simulink model "TareaIntegradora"  (R2023b)
settings: Solver=VariableStepAuto  StartTime=0.0  StopTime=9  FixedStep=0.001  RelTol=1e-3  EnableMultiTasking=on
InitFcn:
  | L= 0.000938
  | J=0.0072
  | B=0.000389
  | b=B
  | R=5.2
  | km=0.5931
  | K=km
  | Radio=0.05
settings Model: ExtModeTrigDuration=2  Creator=jaime  LastModifiedBy=jaime
settings OptimizationCC: EnhancedBackFolding=on  PassReuseOutputArgsAs=Individual arguments  ZeroExternalMemoryAtStartup=off  ZeroInternalMemoryAtStartup=off  MaxStackSize=64  OptimizeBlockOrder=speed  DifferentSizesBufferReuse=on  OptimizationCustomize=off  EfficientTunableParamExpr=on
settings DebuggingCC: ParameterTunabilityLossMsg=error
settings HardwareCC: ProdBitPerInt=16  ProdBitPerPointer=16  ProdBitPerSizeT=16  ProdBitPerPtrDiffT=16  ProdLargestAtomicFloat=None  ProdWordSize=8  ProdHWDeviceType=Atmel->AVR  UseEmbeddedCoderFeatures=off
settings SFSimCC: MATLABDynamicMemAlloc=off
settings RTWCC: Description=Embedded Coder  SystemTargetFile=ert.tlc  HardwareBoard=Arduino Mega 2560  TemplateMakefile=ert_default_tmf  Toolchain=Arduino AVR  BuildConfiguration=Faster Runs
settings CodeAppCC: ForceParamTrailComments=on  IgnoreCustomStorageClasses=off  OperatorAnnotations=on  SimulinkDataObjDesc=on  SFDataObjDesc=on  InsertBlockDesc=on
settings ERTTargetCC: SupportContinuousTime=on  SupportNonInlinedSFcns=on  SupportVariableSizeSignals=on  ExtModeTransport=3  ExtModeStaticAlloc=on  ExtModeAutomaticAllocSize=off  ExtModeStaticAllocSize=2048  ExtModeMexFile=ext_xcp  ExtModeIntrfLevel=Level2 - Open

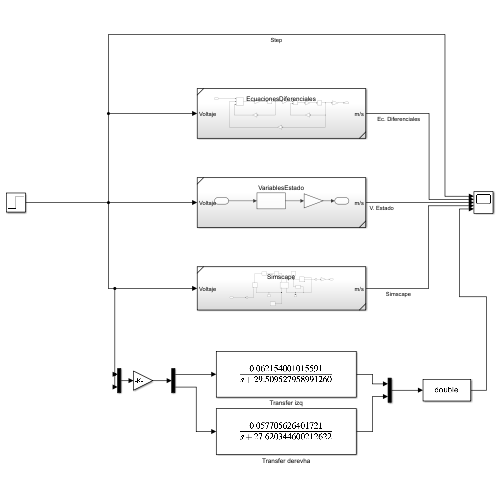
[thumbnail: Simulink's stored preview of the top-level diagram]
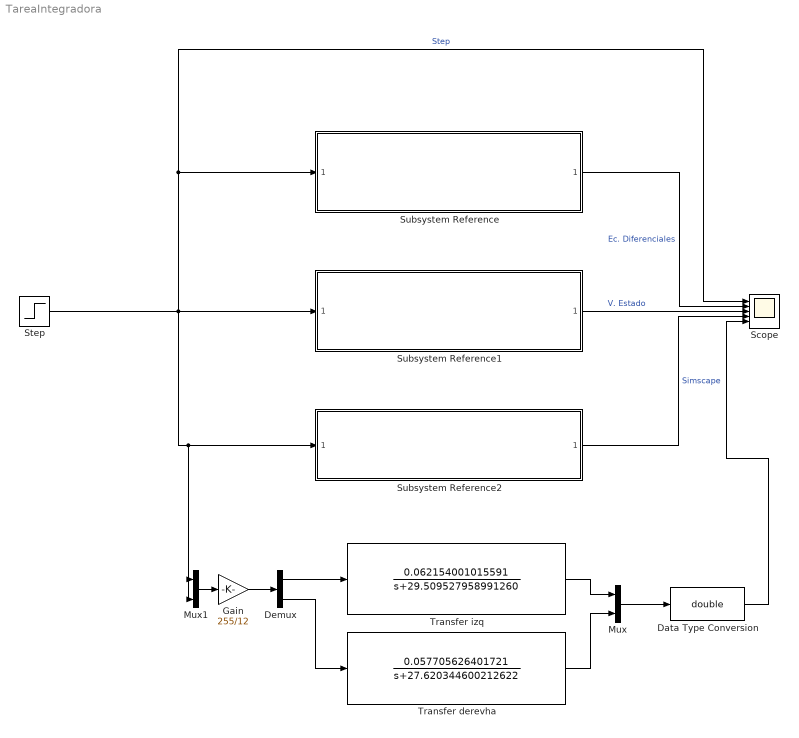
== system TareaIntegradora ==
  Data Type Conversion : DataTypeConversion  OutDataTypeStr=double  SaturateOnIntegerOverflow=off  RndMeth=Floor
  Demux : Demux  Outputs=2
  Gain : Gain  Gain=255/12
  Mux : Mux  Inputs=2
  Mux1 : Mux  Inputs=2
  Scope : Scope  NumInputPorts=5
  Step : Step  After=11.8  SampleTime=0
  Subsystem Reference : Subsystem  ReferencedSubsystem=EcuacionesDiferenciales
  Subsystem Reference1 : Subsystem  ReferencedSubsystem=VariablesEstado
  Subsystem Reference2 : Subsystem  ReferencedSubsystem=Simscape
  Transfer derevha : TransferFcn  Numerator=0.057705626401721  Denominator=[1,27.620344600212622]
  Transfer izq : TransferFcn  Numerator=0.062154001015591  Denominator=[1,29.509527958991260]
  wires:
  Subsystem Reference/1 -> Scope/2  "Ec. Diferenciales"
  Step/1 -> Subsystem Reference/1, Scope/1, Mux1/2, Mux1/1, Subsystem Reference2/1, Subsystem Reference1/1  "Step"
  Subsystem Reference2/1 -> Scope/4  "Simscape"
  Subsystem Reference1/1 -> Scope/3  "V. Estado"
  Transfer izq/1 -> Mux/1
  Transfer derevha/1 -> Mux/2
  Mux/1 -> Data Type Conversion/1
  Data Type Conversion/1 -> Scope/5
  Demux/1 -> Transfer izq/1
  Demux/2 -> Transfer derevha/1
  Gain/1 -> Demux/1
  Mux1/1 -> Gain/1
